simulink model "si3_int_statt_diff"  (R2021b)
settings: Solver=VariableStepAuto  StartTime=0.0  StopTime=10  RelTol=1e-3
settings Model: Creator=Bob  LastModifiedBy=sar
settings SolverCC: AlgebraicLoopSolver=TrustRegion
settings DataIOCC: ReturnWorkspaceOutputs=off
settings DebuggingCC: SFMachineParentedDataDiag=warning  ArithmeticOperatorsInVariantConditions=warning
settings SFSimCC: CustomCodeUndefinedFunction=UseInterfaceOnly

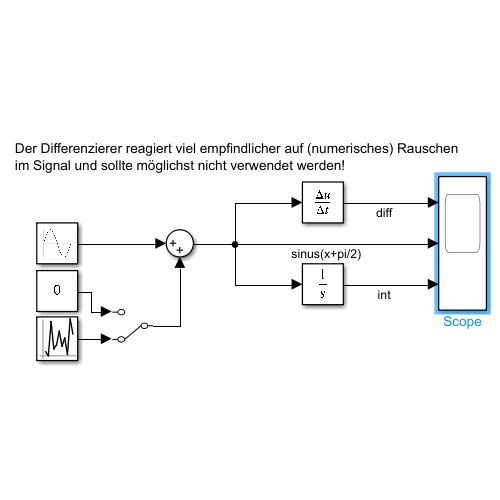
[thumbnail: Simulink's stored preview of the top-level diagram]
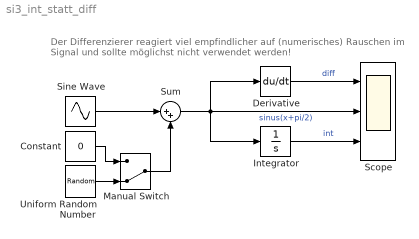
== system si3_int_statt_diff ==
  note: Der Differenzierer reagiert viel empfindlicher auf (numerisches) Rauschen im Signal und sollte möglichst nicht verwendet werden!
  Constant : Constant  Value=0
  Derivative : Derivative
  Integrator : Integrator
  Manual Switch : ManualSwitch  CurrentSetting=0
  Scope : Scope  NumInputPorts=3
  Sine Wave : Sin  Phase=pi/2  SampleTime=0
  Sum : Sum  Inputs=|++
  Uniform Random Number : UniformRandomNumber  Minimum=-0.025  Maximum=0.025  SampleTime=0.1
  wires:
  Integrator/1 -> Scope/3  "int"
  Derivative/1 -> Scope/1  "diff"
  Sum/1 -> Integrator/1, Scope/2, Derivative/1  "sinus(x+pi/2)"
  Sine Wave/1 -> Sum/1
  Uniform Random Number/1 -> Manual Switch/2
  Manual Switch/1 -> Sum/2
  Constant/1 -> Manual Switch/1
